simulink model "MotorIsOverMaxPosChk"  (R2018b)
settings: Solver=FixedStepDiscrete  StartTime=0.0  StopTime=10.0  FixedStep=0.01  RelTol=1e-3
settings Model: Creator=sn2xws  LastModifiedBy=sn2xws
settings DataIOCC: SaveFormat=StructureWithTime
settings OptimizationCC: DefaultParameterBehavior=Inlined  EnhancedBackFolding=on  PassReuseOutputArgsAs=Individual arguments  ZeroExternalMemoryAtStartup=off  ZeroInternalMemoryAtStartup=off  OptimizeBlockOrder=speed  DifferentSizesBufferReuse=on  OptimizationCustomize=off
settings DebuggingCC: ParameterTunabilityLossMsg=error
settings SFSimCC: MATLABDynamicMemAlloc=off
settings RTWCC: SystemTargetFile=autosar.tlc  GenCodeOnly=on  TemplateMakefile=ert_default_tmf  Description=AUTOSAR  GenerateReport=on  IncludeHyperlinkInReport=on  LaunchReport=on  GenerateTraceInfo=on  GenerateTraceReport=on  GenerateTraceReportSl=on  GenerateTraceReportSf=on  GenerateTraceReportEml=on  GenerateCodeMetricsReport=on
settings CodeAppCC: ForceParamTrailComments=on  IgnoreCustomStorageClasses=off  OperatorAnnotations=on  SimulinkDataObjDesc=on  SFDataObjDesc=on  InsertBlockDesc=on
settings STFCustomTargetCC: TargetLangStandard=C99 (ISO)  MultiwordLength=256  ParMdlRefBuildCompliant=on  CompOptLevelCompliant=on  IncludeMdlTerminateFcn=off  CombineOutputUpdateFcns=on  SuppressErrorStatus=on  ERTCustomFileBanners=on  SupportNonFinite=off  SupportComplex=off  SupportContinuousTime=off  SupportNonInlinedSFcns=off  RemoveResetFunc=on  MATLABClassNameForMDSCustomization=Simulink.SoftwareTarget.ERTCustomization  AutosarCompliant=on  UseToolchainInfoCompliant=on  LookupTableObjectStructAxisOrder=2,1,3,4,...  LUTObjectStructOrderEvenSpacing=Size,Table,Breakpoints  SystemTargetFile=autosar.tlc
settings ERTTargetCC: TargetLangStandard=C99 (ISO)  ConcurrentExecutionCompliant=off  IncludeMdlTerminateFcn=off  SuppressErrorStatus=on  SupportNonFinite=off  SupportComplex=off  ModelStepFunctionPrototypeControlCompliant=off  CPPClassGenCompliant=off  AutosarCompliant=on  LookupTableObjectStructAxisOrder=2,1,3,4,...  LUTObjectStructOrderEvenSpacing=Size,Table,Breakpoints  InlinedParameterPlacement=NonHierarchical  ERTCustomFileTemplate=example_file_process.tlc  ERTFilePackagingFormat=Compact

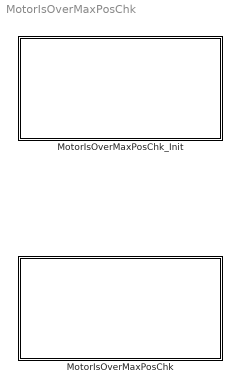
== system MotorIsOverMaxPosChk ==
  MotorIsOverMaxPosChk : Subsystem
  MotorIsOverMaxPosChk_Init : Subsystem

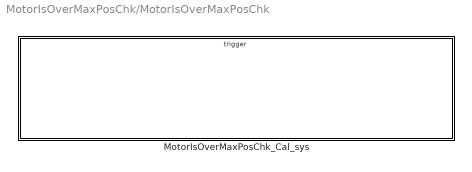
== system MotorIsOverMaxPosChk/MotorIsOverMaxPosChk ==
  MotorIsOverMaxPosChk_Cal_sys : Subsystem

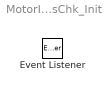
== system MotorIsOverMaxPosChk/MotorIsOverMaxPosChk_Init ==
  Event Listener : EventListener  EventName=reset

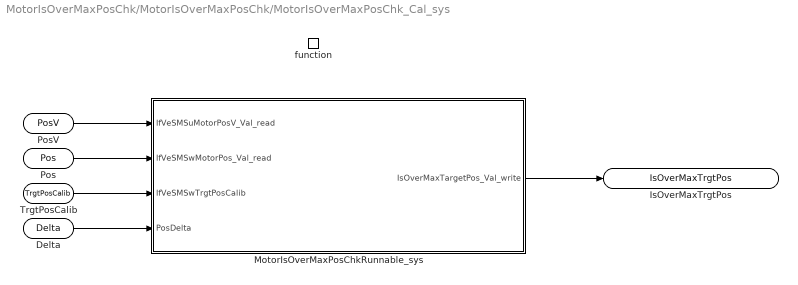
== system MotorIsOverMaxPosChk/MotorIsOverMaxPosChk/MotorIsOverMaxPosChk_Cal_sys ==
  function : TriggerPort  TriggerType=function-call  IsSimulinkFunction=on  FunctionName=MotorIsOverMaxPosChk_Cal  VariantControl=(inherit)
  MotorIsOverMaxPosChkRunnable_sys : Subsystem
  PosV : ArgIn  OutDataTypeStr=boolean  ArgumentName=PosV
  Pos : ArgIn  Port=2  OutDataTypeStr=uint16  ArgumentName=Pos
  TrgtPosCalib : ArgIn  Port=3  OutDataTypeStr=uint16  PortDimensions=3  ArgumentName=TrgtPosCalib
  Delta : ArgIn  Port=4  OutDataTypeStr=uint16  ArgumentName=Delta
  IsOverMaxTrgtPos : ArgOut  OutDataTypeStr=boolean  ArgumentName=IsOverMaxTrgtPos
  wires:
  PosV/1 -> MotorIsOverMaxPosChkRunnable_sys/1(IfVeSMSuMotorPosV_Val_read)
  Pos/1 -> MotorIsOverMaxPosChkRunnable_sys/2(IfVeSMSwMotorPos_Val_read)
  TrgtPosCalib/1 -> MotorIsOverMaxPosChkRunnable_sys/3(IfVeSMSwTrgtPosCalib)
  Delta/1 -> MotorIsOverMaxPosChkRunnable_sys/4(PosDelta)
  MotorIsOverMaxPosChkRunnable_sys/1(IsOverMaxTargetPos_Val_write) -> IsOverMaxTrgtPos/1

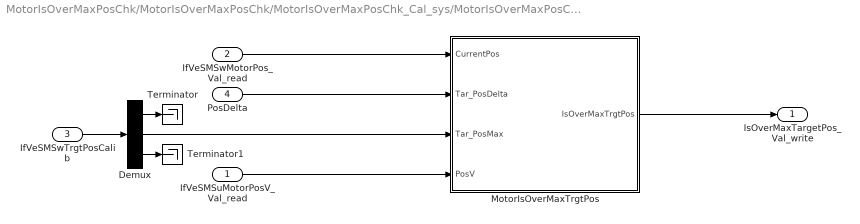
== system MotorIsOverMaxPosChk/MotorIsOverMaxPosChk/MotorIsOverMaxPosChk_Cal_sys/MotorIsOverMaxPosChkRunnable_sys ==
  IfVeSMSuMotorPosV_Val_read : Inport
  IfVeSMSwMotorPos_Val_read : Inport  Port=2
  IfVeSMSwTrgtPosCalib : Inport  Port=3
  PosDelta : Inport  Port=4
  Demux : Demux  Outputs=3
  MotorIsOverMaxTrgtPos : Subsystem
  Terminator : Terminator
  Terminator1 : Terminator
  IsOverMaxTargetPos_Val_write : Outport
      settings: EnsureOutportIsVirtual=on
  wires:
  IfVeSMSuMotorPosV_Val_read/1 -> MotorIsOverMaxTrgtPos/4(PosV)
  IfVeSMSwMotorPos_Val_read/1 -> MotorIsOverMaxTrgtPos/1(CurrentPos)
  MotorIsOverMaxTrgtPos/1(IsOverMaxTrgtPos) -> IsOverMaxTargetPos_Val_write/1
  PosDelta/1 -> MotorIsOverMaxTrgtPos/2(Tar_PosDelta)
  IfVeSMSwTrgtPosCalib/1 -> Demux/1
  Demux/2 -> MotorIsOverMaxTrgtPos/3(Tar_PosMax)
  Demux/1 -> Terminator/1
  Demux/3 -> Terminator1/1

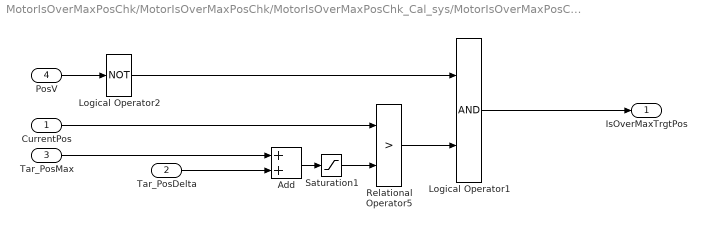
== system MotorIsOverMaxPosChk/MotorIsOverMaxPosChk/MotorIsOverMaxPosChk_Cal_sys/MotorIsOverMaxPosChkRunnable_sys/MotorIsOverMaxTrgtPos ==
  CurrentPos : Inport
  Tar_PosDelta : Inport  Port=2
  Tar_PosMax : Inport  Port=3
  PosV : Inport  Port=4
  Add : Sum
  Logical Operator1 : Logic  AllPortsSameDT=off  OutDataTypeStr=boolean
  Logical Operator2 : Logic  Operator=NOT  AllPortsSameDT=off  OutDataTypeStr=boolean
  Relational Operator5 : RelationalOperator  Operator=>  OutDataTypeStr=boolean  RndMeth=Simplest
  Saturation1 : Saturate  UpperLimit=4095  LowerLimit=0
  IsOverMaxTrgtPos : Outport
  wires:
  Tar_PosDelta/1 -> Add/2
  Add/1 -> Saturation1/1
  Saturation1/1 -> Relational Operator5/2
  CurrentPos/1 -> Relational Operator5/1
  Tar_PosMax/1 -> Add/1
  PosV/1 -> Logical Operator2/1
  Logical Operator2/1 -> Logical Operator1/1
  Relational Operator5/1 -> Logical Operator1/2
  Logical Operator1/1 -> IsOverMaxTrgtPos/1
